simulink model "prototype_dashboard"  (R2024b)
settings: Solver=FixedStepAuto  StartTime=0.0  StopTime=inf  RelTol=1e-3  EnableMultiTasking=on
libraries: stm32f4xxblockslib x7, simulink x2
settings Model: STM32="{\"DigitalPortRead\":[{\"ID\":\"stm32test:431\"},{\"ID\":\"stm32test:432\"},{\"ID\":\"stm32test:483\"},{\"ID\":\"stm32test:484\"},{\"ID\":\"stm32test:504\"},{\"ID\":\"stm32test:505\"},{\"ID\":\"stm32test:895\"},{\"ID\":\"stm32test:896\"},{\"ID\":\"stm32test:1060\"},{\"ID\":\"stm32test:1031\"},{\"ID\":\"stm32test:1185\"},{\"ID\":\"stm32test:1186\"},{\"ID\":\"stm32test:1192\"},{\"ID\":\"stm32test:1193\"},{\"ID\":\"stm32test:1194\"},{\"ID\":\"stm32test:1195\"},{\"ID\":\"stm32test:1388:438\"},{\"ID\":\"stm32test:1590\"}],\"PWMOutput\":[{\"ID\":\"stm32test:6\"},{\"ID\":\"stm32test:8\"},{\"ID\":\"stm32test:1305\"},{\"ID\":\"stm32test:1306\"},{\"ID\":\"stm32test:1562\"}],\"DigitalPortWrite\":[{\"ID\":\"stm32test:1295\"},{\"ID\":\"stm32test:1307\"},{\"ID\":\"stm32test:1481\"},{\"ID\":\"stm32test:1482\"}],\"TimerCapture\":[{\"ID\":\"stm32test:166\"},{\"ID\":\"stm32test:836\"},{\"ID\":\"stm32test:1074\"},{\"ID\":\"stm32test:1045\"},{\"ID\":\"stm32test:1103\"},{\"ID\":\"stm32test:1388:414\"},{\"ID\":\"stm32test:1132\"},{\"ID\":\"stm32test:1468:414\"},{\"ID\":\"stm32test:1542\"}],\"HardwareInterrupt\":[{\"ID\":\"stm32test:102\"},{\"ID\":\"stm32test:1388:418\"}]}"  Creator=Tarsoly  LastModifiedBy=Asus
settings OptimizationCC: BlockReduction=off  BooleanDataType=off  EnhancedBackFolding=on  PassReuseOutputArgsAs=Individual arguments  ZeroExternalMemoryAtStartup=off  ZeroInternalMemoryAtStartup=off  MaxStackSize=512  OptimizeBlockOrder=speed  DifferentSizesBufferReuse=on  OptimizationCustomize=off  EfficientTunableParamExpr=on
settings DebuggingCC: SaveWithParameterizedLinksMsg=none  MergeDetectMultiDrivingBlocksExec=none  SignalResolutionControl=TryResolveAllWithWarning  ParameterTunabilityLossMsg=error
settings HardwareCC: ProdBitPerPointer=32  ProdBitPerSizeT=32  ProdBitPerPtrDiffT=32  ProdLargestAtomicInteger=Long  ProdLargestAtomicFloat=Double  ProdWordSize=32  ProdHWDeviceType=ARM Compatible->ARM Cortex-M  TargetLargestAtomicInteger=Long  TargetLargestAtomicFloat=Double  TargetIntDivRoundTo=Zero  TargetEndianess=LittleEndian  TargetHWDeviceType=ARM Compatible->ARM Cortex-M
settings ModelReferenceCC: PropagateSignalLabelsOutOfModel=off
settings SFSimCC: SimCustomHeaderCode="#include \"SensorActuator.h\""  SimCustomInitializer=Timer_Init_Custom();  SimUserSources=SensorActuator.c  SimUserDefines=STM32F411xE  MATLABDynamicMemAlloc=off
settings SFSimCC: SimUserIncludeDirs=|
  | D:\BME\Hetedik_felev\Szakdoga\Matlab\C_kod
  | D:\CubeMXProjectFiles\tanfolyamrobot\Core\Inc
  | D:\CubeMXProjectFiles\tanfolyamrobot\Drivers\STM32F4xx_HAL_Driver\Inc
  | D:\CubeMXProjectFiles\tanfolyamrobot\Drivers\CMSIS\Device\ST\STM32F4xx\Include
  | D:\CubeMXProjectFiles\tanfolyamrobot\Drivers\CMSIS\Include
settings RTWCC: Description=Embedded Coder  SystemTargetFile=ert.tlc  HardwareBoard=STM32F4xx Based  TemplateMakefile=ert_default_tmf  RTWUseSimCustomCode=on  CustomHeaderCode="#include \"SensorActuator.h\""  CustomSource=SensorActuator.c  CustomDefine=STM32F411xE  CustomInitializer=Timer_Init_Custom();  Toolchain=GNU Tools for ARM Embedded Processors
settings RTWCC: CustomInclude=|
  | D:\BME\Hetedik_felev\Szakdoga\Matlab\C_kod
  | D:\CubeMXProjectFiles\tanfolyamrobot\Core\Inc
  | D:\CubeMXProjectFiles\tanfolyamrobot\Drivers\STM32F4xx_HAL_Driver\Inc
  | D:\CubeMXProjectFiles\tanfolyamrobot\Drivers\CMSIS\Device\ST\STM32F4xx\Include
  | D:\CubeMXProjectFiles\tanfolyamrobot\Drivers\CMSIS\Include
settings CodeAppCC: ForceParamTrailComments=on  IgnoreCustomStorageClasses=off  OperatorAnnotations=on  SimulinkDataObjDesc=on  SFDataObjDesc=on  InsertBlockDesc=on
settings ERTTargetCC: TargetLangStandard=C99 (ISO)  CodeReplacementLibrary=ARM Cortex-M  ExtModeTransport=3  ExtModeStaticAlloc=on  ExtModeStaticAllocSize=2048  ExtModeMexFile=ext_xcp  ExtModeIntrfLevel=Level2 - Open  InlinedParameterPlacement=Hierarchical

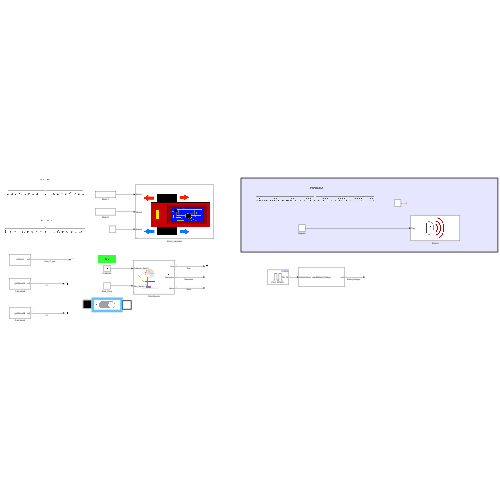
[thumbnail: Simulink's stored preview of the top-level diagram]
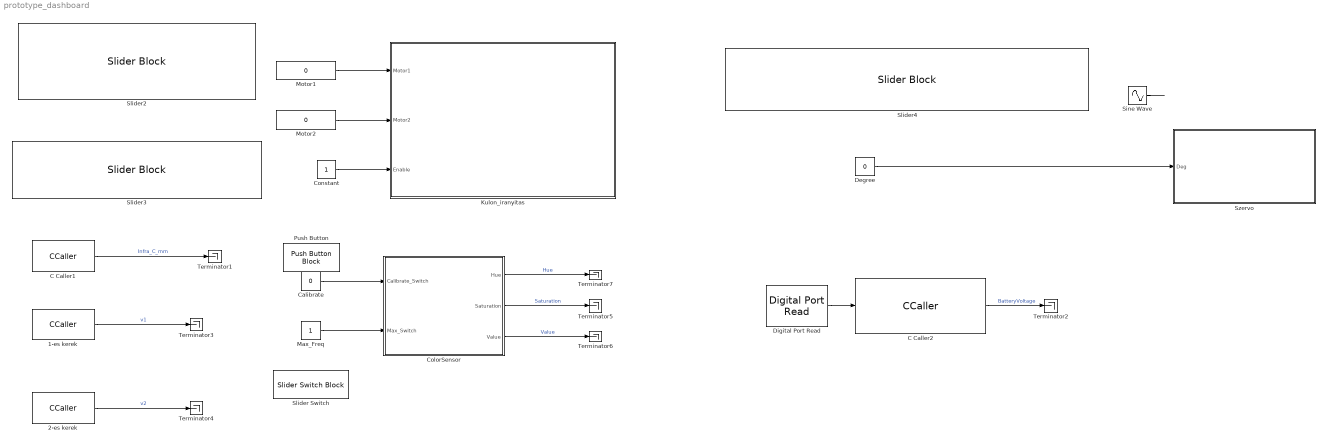
== system prototype_dashboard ==
  1-es kerek : CCaller  FunctionName=getSpeedA  PortSpecificationStruct="%)30     .    & (   8    (     @         %    \"     $    !     0         %  0 \"0    $    _    07)G3F%M90  4&]R=$YA;64 4V-O<&4     26YD97@     5'EP90      4VEZ90      27-';&]B86P   X    P    !@    @    $          4    (     0    ,    !         !   P!O=70 #@   #     &    \"     0         !0    @    !     P    $         $  # &]U=  .    .     8    (    !          %    \"     $    &     0         0    !@   $]U='!U=   #@   #@    &    \"     8         !0    @    !     0    $         \"0    @               X    X    !@    @    $          4    (     0    8    !         !     &    9&]U8FQE   .    ,     8    (    !          %    \"     $    !     0         0  $ ,0    X    P    !@    @    ) @        4    (     0    $    !          (  0"  SampleTime=0.02
  2-es kerek : CCaller  FunctionName=getSpeedB  PortSpecificationStruct="%)30     .    & (   8    (     @         %    \"     $    !     0         %  0 \"0    $    _    07)G3F%M90  4&]R=$YA;64 4V-O<&4     26YD97@     5'EP90      4VEZ90      27-';&]B86P   X    P    !@    @    $          4    (     0    ,    !         !   P!O=70 #@   #     &    \"     0         !0    @    !     P    $         $  # &]U=  .    .     8    (    !          %    \"     $    &     0         0    !@   $]U='!U=   #@   #@    &    \"     8         !0    @    !     0    $         \"0    @               X    X    !@    @    $          4    (     0    8    !         !     &    9&]U8FQE   .    ,     8    (    !          %    \"     $    !     0         0  $ ,0    X    P    !@    @    ) @        4    (     0    $    !          (  0"  SampleTime=0.02
  C Caller1 : CCaller  FunctionName=infrared  PortSpecificationStruct="%)30     .    & (   8    (     @         %    \"     $    !     0         %  0 \"0    $    _    07)G3F%M90  4&]R=$YA;64 4V-O<&4     26YD97@     5'EP90      4VEZ90      27-';&]B86P   X    P    !@    @    $          4    (     0    ,    !         !   P!O=70 #@   #     &    \"     0         !0    @    !     P    $         $  # &]U=  .    .     8    (    !          %    \"     $    &     0         0    !@   $]U='!U=   #@   #@    &    \"     8         !0    @    !     0    $         \"0    @               X    X    !@    @    $          4    (     0    8    !         !     &    =6EN=#,R   .    ,     8    (    !          %    \"     $    !     0         0  $ ,0    X    P    !@    @    ) @        4    (     0    $    !          (  0"  SampleTime=0.02
  C Caller2 : CCaller  FunctionName=readBatteryVoltage  PortSpecificationStruct="%)30     .    V ,   8    (     @         %    \"     (    !     0         %  0 \"0    $    _    07)G3F%M90  4&]R=$YA;64 4V-O<&4     26YD97@     5'EP90      4VEZ90      27-';&]B86P   X    P    !@    @    $          4    (     0    ,    !         !   P!O=70 #@   #     &    \"     0         !0    @    !     P    $         $  # &]U=  .    .     8    (    !          %    \"     $    &     0         0    !@   $]U='!U=   #@   #@    &    \"     8         !0    @    !     0    $         \"0    @               X    X    !@    @    $          4    (     0    8    !         !     &    =6EN=#$V   .    ,     8    (    !          %    \"     $    !     0         0  $ ,0    X    P    !@    @    ) @        4    (     0    $    !          (  0      #@   $     &    \"     0         !0    @    !    \"P    $         $     L   !B=71T;VY686QU90      #@   $     &    \"     0         !0    @    !    \"P    $         $     L   !B=71T;VY686QU90      #@   #@    &    \"     0         !0    @    !    !0    $         $     4   !);G!U=     X    X    !@    @    &          4    (     0    $    !          D    (               .    .     8    (    !          %    \"     $    '     0         0    !P   &)O;VQE86X #@   #     &    \"     0         !0    @    !     0    $         $  ! #$    .    ,     8    (    \"0(        %    \"     $    !     0         \"  $"  SampleTime=1
  Calibrate : Constant  Value=0
  ColorSensor : Subsystem
      mask DialogControl DescTextVar Prompt: This subsystem is for measuring the color of the ground beneath the robot.
      mask Display: image('Mask5_szin2.png', [20,20,20,20,100,100]);
  Constant : Constant
  Degree : Constant  Value=0
  Digital Port Read : stm32f4xxblockslib/Digital Port Read  PortName=GPIOA  PinNumber=[15]  ReadOperation=on  IOAsArray=off  SampleTime=1  EnableSimPort=off  hoistedMaskSrc=ECSoC/ECSimCodegen/Digital Port Read
  Kulon_iranyitas : Subsystem
      mask DialogControl Control2 Prompt: This block is meant for when you want to control the wheels independent of eachother. It can control the wheels with (-99;99) signals.
      mask Display: image('Maszk4_kulon_kerek.png', [25,25,5,0,100,100]);
  Max_Freq : Constant
  Motor1 : Constant  Value=0
  Motor2 : Constant  Value=0
  Push Button : PushButtonBlock  ButtonText=Calibrate  OffValue=0.000000
  Sine Wave : Sin  Amplitude=90  Frequency=pi  SampleTime=0.02
  Slider Switch : SliderSwitchBlock  LabelPosition=Hide
      settings: Values={{'Off', 'On'}, [0 1]}
  Slider2 : SliderBlock  ScaleMin=-99  ScaleMax=99
  Slider3 : SliderBlock  ScaleMin=-99  ScaleMax=99
  Slider4 : SliderBlock  ScaleMin=-90  ScaleMax=90
  Szervo : Subsystem
      mask Display: image('Mask6_Szervo.png', [30,10,30,10,100,100]);
  Terminator{1..7} (7 alike) : Terminator
  wires:
  Constant/1 -> Kulon_iranyitas/3(Enable)
  Motor1/1 -> Kulon_iranyitas/1(Motor1)
  Motor2/1 -> Kulon_iranyitas/2(Motor2)
  C Caller1/1 -> Terminator1/1  "Infra_C_mm"
  C Caller2/1 -> Terminator2/1  "BatteryVoltage"
  Digital Port Read/1 -> C Caller2/1
  2-es kerek/1 -> Terminator4/1  "v2"
  1-es kerek/1 -> Terminator3/1  "v1"
  Sine Wave/1 -> ?
  ColorSensor/1(Hue) -> Terminator7/1  "Hue"
  ColorSensor/2(Saturation) -> Terminator5/1  "Saturation"
  ColorSensor/3(Value) -> Terminator6/1  "Value"
  Degree/1 -> Szervo/1(Deg)
  Calibrate/1 -> ColorSensor/1(Calibrate_Switch)
  Max_Freq/1 -> ColorSensor/2(Max_Switch)

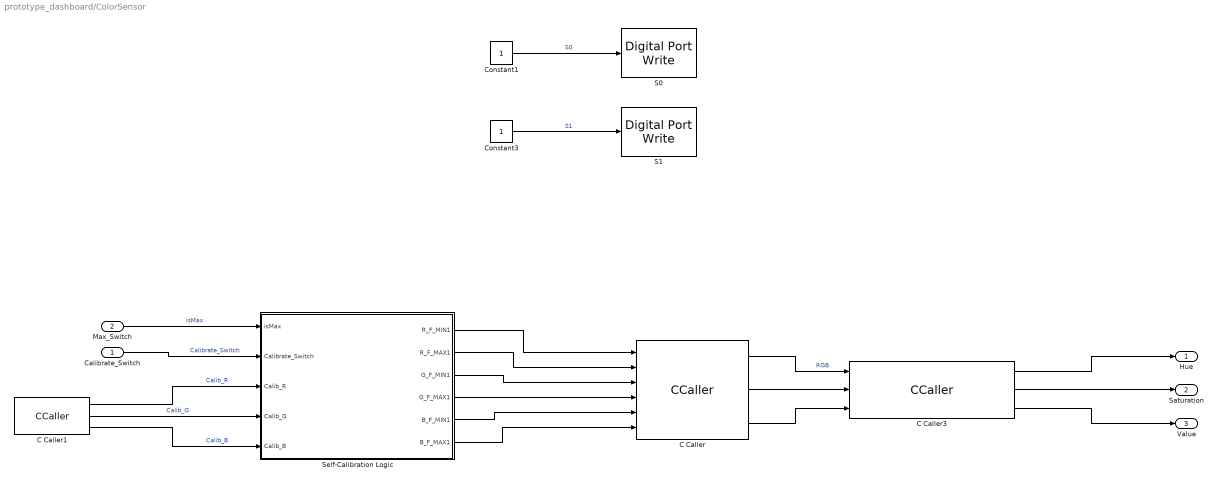
== system prototype_dashboard/ColorSensor ==
  Calibrate_Switch : Inport
  Max_Switch : Inport  Port=2
  C Caller : CCaller  FunctionName=getRGB  PortSpecificationStruct="%)30     .    > \\   8    (     @         %    \"     D    !     0         %  0 \"0    $    _    07)G3F%M90  4&]R=$YA;64 4V-O<&4     26YD97@     5'EP90      4VEZ90      27-';&]B86P   X    P    !@    @    $          4    (     0    $    !         !   0!2    #@   #     &    \"     0         !0    @    !     0    $         $  ! %(    .    .     8    (    !          %    \"     $    &     0         0  ...(+4961 chars)"  SampleTime=0.02
  C Caller1 : CCaller  FunctionName=calibrateRGB  PortSpecificationStruct="%)30     .    6 4   8    (     @         %    \"     ,    !     0         %  0 \"0    $    _    07)G3F%M90  4&]R=$YA;64 4V-O<&4     26YD97@     5'EP90      4VEZ90      27-';&]B86P   X    P    !@    @    $          4    (     0    $    !         !   0!2    #@   #     &    \"     0         !0    @    !     0    $         $  ! %(    .    .     8    (    !          %    \"     $    &     0         0    !@   $]U='!U=   #@   #@    &    \"     8         !0    @    !     0    $         \"0    @               X    X    !@    @    $          4    (     0    8    !         !     &    =6EN=#$V   .    ,     8    (    !          %    \"     $    !     0         0  $ ,0    X    P    !@    @    ) @        4    (     0    $    !          (  0      #@   #     &    \"     0         !0    @    !     0    $         $  ! $<    .    ,     8    (    !          %    \"     $    !     0         0  $ 1P    X    X    !@    @    $          4    (     0    8    !         !     &    3W5T<'5T   .    .     8    (    !@         %    \"     $    !     0         )    \"            / _#@   #@    &    \"     0         !0    @    !    !@    $         $     8   !U:6YT,38   X    P    !@    @    $          4    (     0    $    !         !   0 Q    #@   #     &    \"     D\"        !0    @    !     0    $          @ !       .    ,     8    (    !          %    \"     $    !     0         0  $ 0@    X    P    !@    @    $          4    (     0    $    !         !   0!\"    #@   #@    &    \"     0         !0    @    !    !@    $         $     8   !/=71P=70   X    X    !@    @    &          4    (     0    $    !          D    (             $ .    .     8    (    !          %    \"     $    &     0         0    !@   '5I;G0Q-@  #@   #     &    \"     0         !0    @    !     0    $         $  ! #$    .    ,     8    (    \"0(        %    \"     $    !     0         \"  $"  SampleTime=0.02
  C Caller3 : CCaller  FunctionName=getHSVfromRGB  PortSpecificationStruct="%)30     .    : H   8    (     @         %    \"     8    !     0         %  0 \"0    $    _    07)G3F%M90  4&]R=$YA;64 4V-O<&4     26YD97@     5'EP90      4VEZ90      27-';&]B86P   X    P    !@    @    $          4    (     0    $    !         !   0!2    #@   #     &    \"     0         !0    @    !     0    $         $  ! %(    .    .     8    (    !          %    \"     $    %     0         0   ...(+3211 chars)"
  Constant1 : Constant
  Constant3 : Constant
  S0 : stm32f4xxblockslib/Digital Port Write  PortName=GPIOC  PinNumber=[12]  ReadOperation=off  IOAsArray=on  EnableSimPort=off  hoistedMaskSrc=ECSoC/ECSimCodegen/Digital Port Write
  S1 : stm32f4xxblockslib/Digital Port Write  PortName=GPIOD  PinNumber=[2]  ReadOperation=off  IOAsArray=on  EnableSimPort=off  hoistedMaskSrc=ECSoC/ECSimCodegen/Digital Port Write
  Self-Calibration Logic : Subsystem
  Hue : Outport
  Saturation : Outport  Port=2
  Value : Outport  Port=3
  wires:
  Constant3/1 -> S1/1  "S1"
  Constant1/1 -> S0/1  "S0"
  C Caller3/1 -> Hue/1
  C Caller3/2 -> Saturation/1
  C Caller3/3 -> Value/1
  C Caller/1 -> C Caller3/1  "RGB"
  C Caller/2 -> C Caller3/2
  C Caller/3 -> C Caller3/3
  Max_Switch/1 -> Self-Calibration Logic/1(isMax)  "isMax"
  Calibrate_Switch/1 -> Self-Calibration Logic/2(Calibrate_Switch)  "Calibrate_Switch"
  C Caller1/1 -> Self-Calibration Logic/3(Calib_R)  "Calib_R"
  C Caller1/2 -> Self-Calibration Logic/4(Calib_G)  "Calib_G"
  C Caller1/3 -> Self-Calibration Logic/5(Calib_B)  "Calib_B"
  Self-Calibration Logic/1(R_F_MIN1) -> C Caller/1
  Self-Calibration Logic/2(R_F_MAX1) -> C Caller/2
  Self-Calibration Logic/3(G_F_MIN1) -> C Caller/3
  Self-Calibration Logic/4(G_F_MAX1) -> C Caller/4
  Self-Calibration Logic/5(B_F_MIN1) -> C Caller/5
  Self-Calibration Logic/6(B_F_MAX1) -> C Caller/6

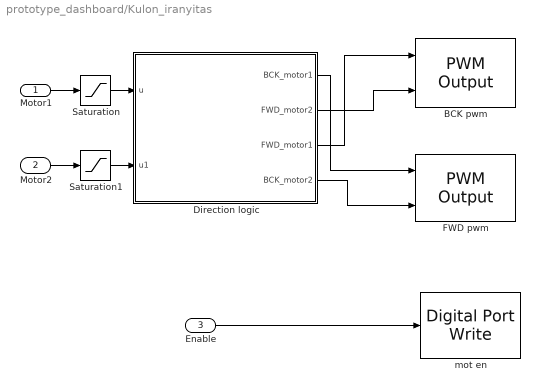
== system prototype_dashboard/Kulon_iranyitas ==
  Motor1 : Inport
  Motor2 : Inport  Port=2
  Enable : Inport  Port=3
  BCK pwm : stm32f4xxblockslib/PWM Output  TimerModule=TIM1  DutycycleUnits=Percentage  EnableChannel1=on  EnableChannel2=on  EnableChannel3=off  EnableChannel4=off  EnableCounterInput=off  EnableMainOutputInput=off  EnableFrequencyInput=off  SetRCAfterCE=off  OutputDirection=off  OutputMainOutputEnableStatus=off  SampleTime=0.1  EnableSimPort=off  EnableUpdateEvent=off  EnableCaptureCompare1Event=off  EnableCaptureCompare2Event=off  EnableCaptureCompare3Event=off  EnableCaptureCompare4Event=off  EnableTriggerEvent=off  EnableBreakEvent=off  ProcessorFamily=STM32F4  hoistedMaskSrc=ECSoC/ECSimCodegen/PWM Output
  Direction logic : Subsystem
  "FWD pwm " : stm32f4xxblockslib/PWM Output  TimerModule=TIM3  DutycycleUnits=Percentage  EnableChannel1=off  EnableChannel2=off  EnableChannel3=on  EnableChannel4=on  EnableCounterInput=off  EnableMainOutputInput=off  EnableFrequencyInput=off  SetRCAfterCE=off  OutputDirection=off  OutputMainOutputEnableStatus=off  SampleTime=0.1  EnableSimPort=off  EnableUpdateEvent=off  EnableCaptureCompare1Event=off  EnableCaptureCompare2Event=off  EnableCaptureCompare3Event=off  EnableCaptureCompare4Event=off  EnableTriggerEvent=off  EnableBreakEvent=off  ProcessorFamily=STM32F4  hoistedMaskSrc=ECSoC/ECSimCodegen/PWM Output
  Saturation : Saturate  UpperLimit=99  LowerLimit=-99
  Saturation1 : Saturate  UpperLimit=99  LowerLimit=-99
  mot en : stm32f4xxblockslib/Digital Port Write  PortName=GPIOC  PinNumber=5  ReadOperation=off  IOAsArray=on  EnableSimPort=off  hoistedMaskSrc=ECSoC/ECSimCodegen/Digital Port Write
  wires:
  Enable/1 -> mot en/1
  Motor1/1 -> Saturation/1
  Motor2/1 -> Saturation1/1
  Direction logic/1(BCK_motor1) -> "FWD pwm "/1
  Direction logic/2(FWD_motor2) -> BCK pwm/2
  Direction logic/3(FWD_motor1) -> BCK pwm/1
  Direction logic/4(BCK_motor2) -> "FWD pwm "/2
  Saturation/1 -> Direction logic/1(u)
  Saturation1/1 -> Direction logic/2(u1)

== system prototype_dashboard/Szervo ==
  Deg : Inport
  PWM Output : stm32f4xxblockslib/PWM Output  TimerModule=TIM11  DutycycleUnits=Percentage  EnableChannel1=on  EnableChannel2=off  EnableChannel3=off  EnableChannel4=off  EnableCounterInput=off  EnableMainOutputInput=off  EnableFrequencyInput=off  SetRCAfterCE=off  OutputDirection=off  OutputMainOutputEnableStatus=off  SampleTime=0.1  EnableSimPort=off  EnableUpdateEvent=off  EnableCaptureCompare1Event=off  EnableCaptureCompare2Event=off  EnableCaptureCompare3Event=off  EnableCaptureCompare4Event=off  EnableTriggerEvent=off  EnableBreakEvent=off  ProcessorFamily=STM32F4  hoistedMaskSrc=ECSoC/ECSimCodegen/PWM Output
  Subsystem2 : Subsystem
  wires:
  Subsystem2/1(f(x)) -> PWM Output/1  "percent"
  Deg/1 -> Subsystem2/1(x)  "x"

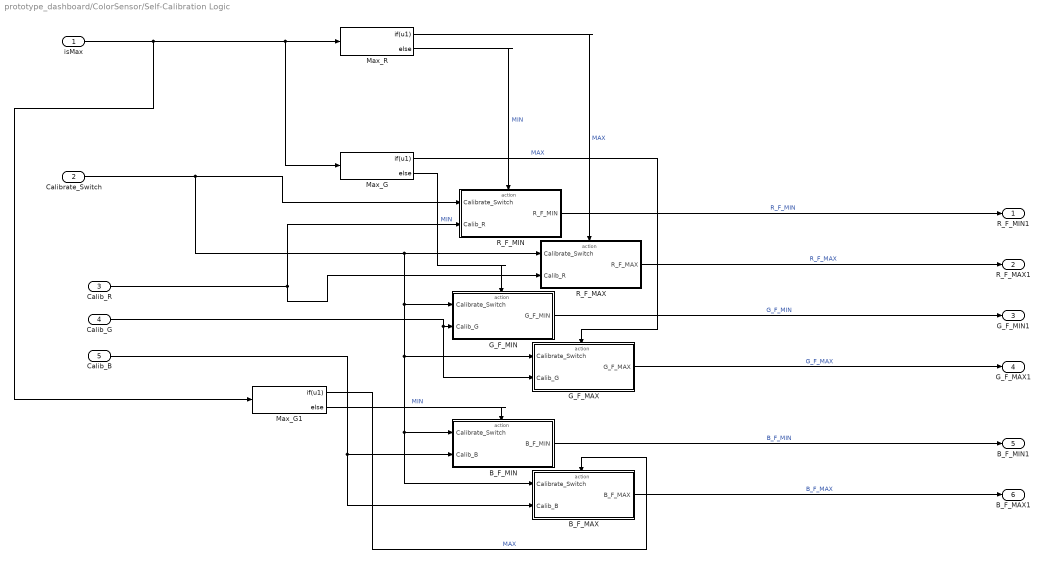
== system prototype_dashboard/ColorSensor/Self-Calibration Logic ==
  isMax : Inport
  Calibrate_Switch : Inport  Port=2
  Calib_R : Inport  Port=3
  Calib_G : Inport  Port=4
  Calib_B : Inport  Port=5
  B_F_MAX : Subsystem  TreatAsAtomicUnit=on
  B_F_MIN : Subsystem  TreatAsAtomicUnit=on
  G_F_MAX : Subsystem  TreatAsAtomicUnit=on
  G_F_MIN : Subsystem  TreatAsAtomicUnit=on
  Max_G : If  IfExpression=u1
  Max_G1 : If  IfExpression=u1
  Max_R : If  IfExpression=u1
  R_F_MAX : Subsystem  TreatAsAtomicUnit=on
  R_F_MIN : Subsystem  TreatAsAtomicUnit=on
  R_F_MIN1 : Outport
  R_F_MAX1 : Outport  Port=2
  G_F_MIN1 : Outport  Port=3
  G_F_MAX1 : Outport  Port=4
  B_F_MIN1 : Outport  Port=5
  B_F_MAX1 : Outport  Port=6
  wires:
  G_F_MIN/1(G_F_MIN) -> G_F_MIN1/1  "G_F_MIN"
  B_F_MAX/1(B_F_MAX) -> B_F_MAX1/1  "B_F_MAX"
  Calib_R/1 -> R_F_MAX/2(Calib_R), R_F_MIN/2(Calib_R)
  Calibrate_Switch/1 -> R_F_MAX/1(Calibrate_Switch), G_F_MIN/1(Calibrate_Switch), B_F_MAX/1(Calibrate_Switch), B_F_MIN/1(Calibrate_Switch), G_F_MAX/1(Calibrate_Switch), R_F_MIN/1(Calibrate_Switch)
  Max_R/1 -> R_F_MAX/Action  "MAX"
  Calib_G/1 -> G_F_MAX/2(Calib_G), G_F_MIN/2(Calib_G)
  G_F_MAX/1(G_F_MAX) -> G_F_MAX1/1  "G_F_MAX"
  Max_R/2 -> R_F_MIN/Action  "MIN"
  isMax/1 -> Max_G/1, Max_R/1, Max_G1/1
  Calib_B/1 -> B_F_MAX/2(Calib_B), B_F_MIN/2(Calib_B)
  B_F_MIN/1(B_F_MIN) -> B_F_MIN1/1  "B_F_MIN"
  R_F_MIN/1(R_F_MIN) -> R_F_MIN1/1  "R_F_MIN"
  R_F_MAX/1(R_F_MAX) -> R_F_MAX1/1  "R_F_MAX"
  Max_G/1 -> G_F_MAX/Action  "MAX"
  Max_G/2 -> G_F_MIN/Action  "MIN"
  Max_G1/1 -> B_F_MAX/Action  "MAX"
  Max_G1/2 -> B_F_MIN/Action  "MIN"

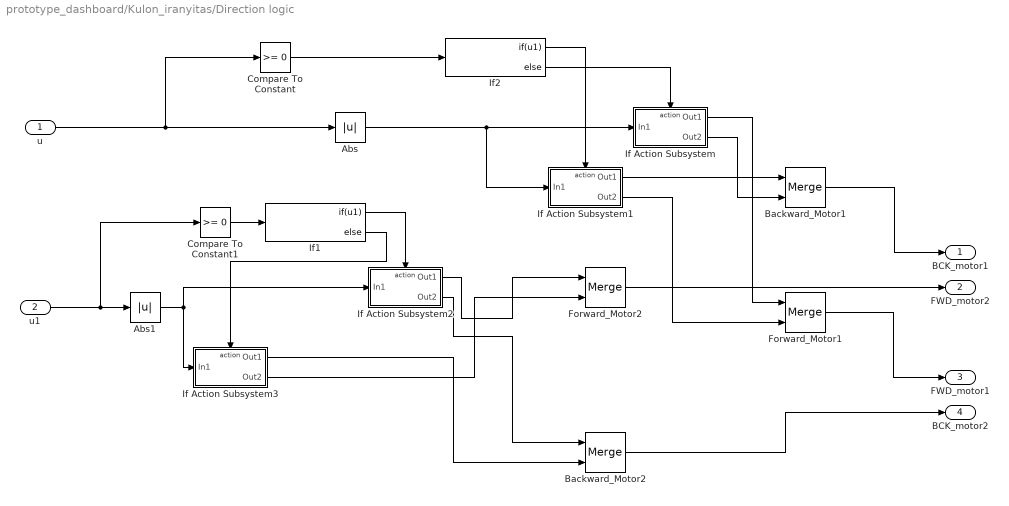
== system prototype_dashboard/Kulon_iranyitas/Direction logic ==
  u : Inport
  u1 : Inport  Port=2
  Abs : Abs  SaturateOnIntegerOverflow=off
  Abs1 : Abs  SaturateOnIntegerOverflow=off
  Backward_Motor1 : Merge
  Backward_Motor2 : Merge
  Compare To Constant : simulink/Logic and Bit Operations/Compare To Constant  relop=>=  const=0  OutDataTypeStr=boolean
  Compare To Constant1 : simulink/Logic and Bit Operations/Compare To Constant  relop=>=  const=0  OutDataTypeStr=boolean
  Forward_Motor1 : Merge
  Forward_Motor2 : Merge
  If Action Subsystem : Subsystem  TreatAsAtomicUnit=on
  If Action Subsystem1 : Subsystem  TreatAsAtomicUnit=on
  If Action Subsystem2 : Subsystem  TreatAsAtomicUnit=on
  If Action Subsystem3 : Subsystem  TreatAsAtomicUnit=on
  If1 : If  IfExpression=u1
  If2 : If  IfExpression=u1
  BCK_motor1 : Outport
  FWD_motor2 : Outport  Port=2
  FWD_motor1 : Outport  Port=3
  BCK_motor2 : Outport  Port=4
  wires:
  Forward_Motor2/1 -> FWD_motor2/1
  If Action Subsystem/1(Out1) -> Forward_Motor1/1
  If Action Subsystem1/1(Out1) -> Backward_Motor1/1
  If Action Subsystem3/2(Out2) -> Forward_Motor2/2
  Compare To Constant/1 -> If2/1
  If Action Subsystem3/1(Out1) -> Backward_Motor2/2
  Abs1/1 -> If Action Subsystem2/1(In1), If Action Subsystem3/1(In1)
  Abs/1 -> If Action Subsystem1/1(In1), If Action Subsystem/1(In1)
  If Action Subsystem/2(Out2) -> Backward_Motor1/2
  u/1 -> Abs/1, Compare To Constant/1
  Backward_Motor2/1 -> BCK_motor2/1
  If1/1 -> If Action Subsystem2/Action
  Compare To Constant1/1 -> If1/1
  u1/1 -> Compare To Constant1/1, Abs1/1
  Backward_Motor1/1 -> BCK_motor1/1
  If1/2 -> If Action Subsystem3/Action
  If Action Subsystem1/2(Out2) -> Forward_Motor1/2
  If Action Subsystem2/1(Out1) -> Forward_Motor2/1
  If Action Subsystem2/2(Out2) -> Backward_Motor2/1
  Forward_Motor1/1 -> FWD_motor1/1
  If2/2 -> If Action Subsystem/Action
  If2/1 -> If Action Subsystem1/Action

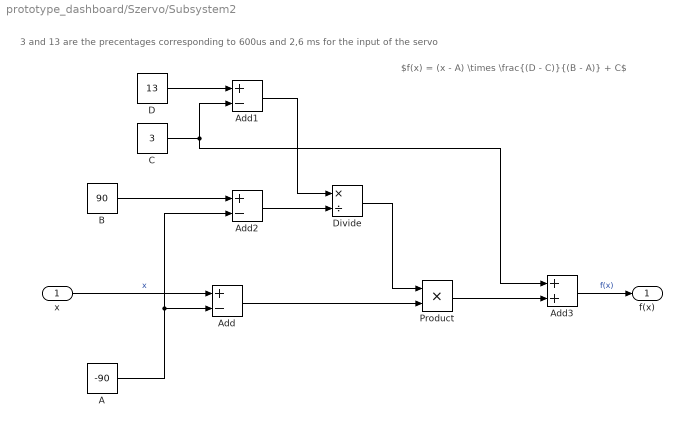
== system prototype_dashboard/Szervo/Subsystem2 ==
  note: 3 and 13 are the precentages corresponding to 600us and 2,6 ms for the input of the servo
  note: $f(x) = (x - A) \times \frac{(D - C)}{(B - A)} + C$
  x : Inport
  A : Constant  Value=-90
  Add : Sum  Inputs=+-
  Add1 : Sum  Inputs=+-
  Add2 : Sum  Inputs=+-
  Add3 : Sum
  B : Constant  Value=90
  C : Constant  Value=3
  D : Constant  Value=13
  Divide : Product  Inputs=*/
  Product : Product
  f(x) : Outport
  wires:
  x/1 -> Add/1  "x"
  A/1 -> Add2/2, Add/2
  Add/1 -> Product/2
  D/1 -> Add1/1
  C/1 -> Add1/2, Add3/1
  Add1/1 -> Divide/1
  Add2/1 -> Divide/2
  B/1 -> Add2/1
  Product/1 -> Add3/2
  Add3/1 -> f(x)/1  "f(x)"
  Divide/1 -> Product/1

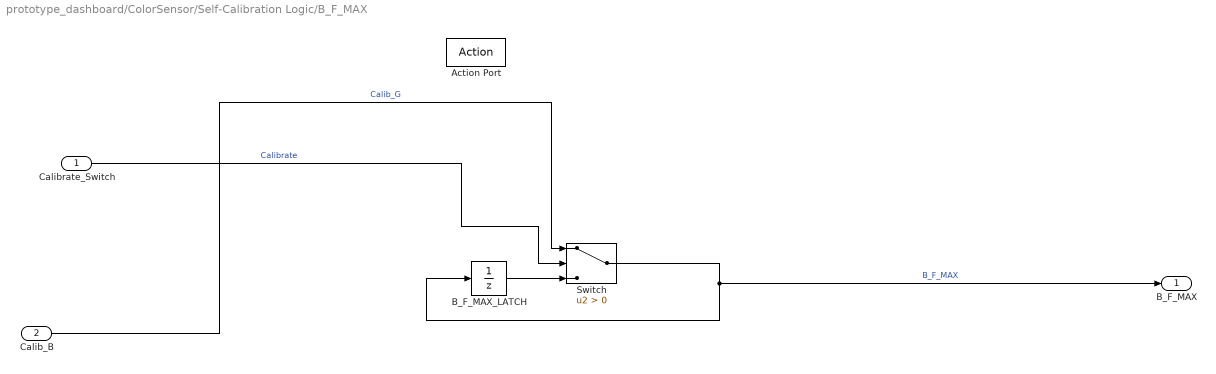
== system prototype_dashboard/ColorSensor/Self-Calibration Logic/B_F_MAX ==
  Calibrate_Switch : Inport
  Calib_B : Inport  Port=2
  Action Port : ActionPort  ActionPortLabel=if(u1)
  B_F_MAX_LATCH : UnitDelay  InitialCondition=18200  SampleTime=-1  HasFrameUpgradeWarning=on
  Switch : Switch  Criteria=u2 > Threshold  SaturateOnIntegerOverflow=off  InputSameDT=off
  B_F_MAX : Outport
  wires:
  Calibrate_Switch/1 -> Switch/2  "Calibrate"
  Calib_B/1 -> Switch/1  "Calib_G"
  Switch/1 -> B_F_MAX_LATCH/1, B_F_MAX/1  "B_F_MAX"
  B_F_MAX_LATCH/1 -> Switch/3

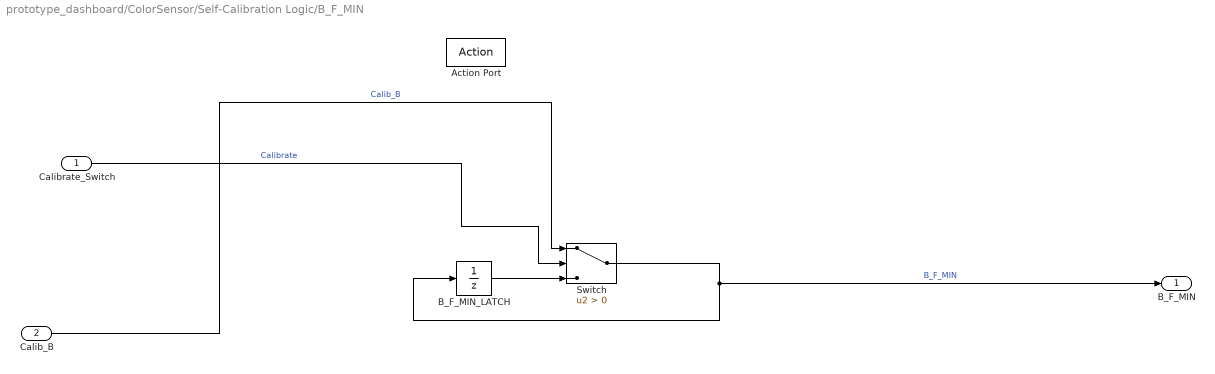
== system prototype_dashboard/ColorSensor/Self-Calibration Logic/B_F_MIN ==
  Calibrate_Switch : Inport
  Calib_B : Inport  Port=2
  Action Port : ActionPort  ActionPortLabel=else
  B_F_MIN_LATCH : UnitDelay  InitialCondition=3200  SampleTime=-1  HasFrameUpgradeWarning=on
  Switch : Switch  Criteria=u2 > Threshold  SaturateOnIntegerOverflow=off  InputSameDT=off
  B_F_MIN : Outport
  wires:
  Calibrate_Switch/1 -> Switch/2  "Calibrate"
  Calib_B/1 -> Switch/1  "Calib_B"
  Switch/1 -> B_F_MIN_LATCH/1, B_F_MIN/1  "B_F_MIN"
  B_F_MIN_LATCH/1 -> Switch/3

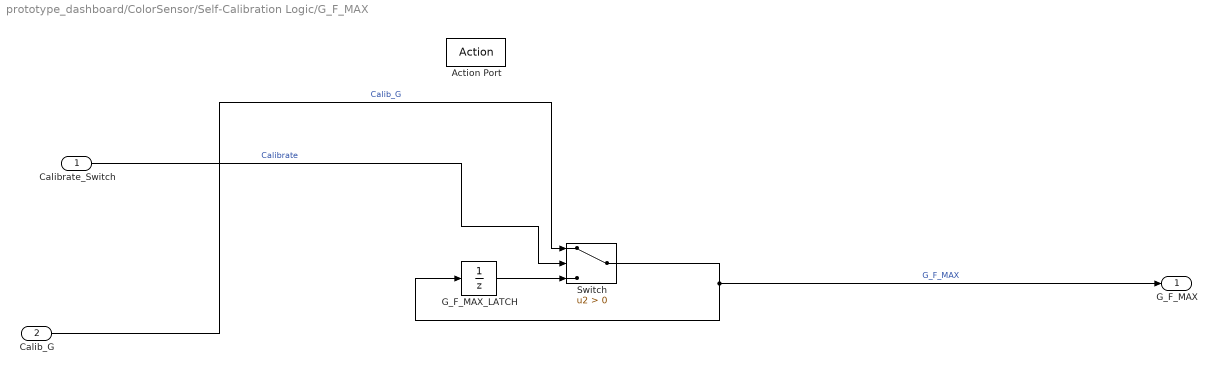
== system prototype_dashboard/ColorSensor/Self-Calibration Logic/G_F_MAX ==
  Calibrate_Switch : Inport
  Calib_G : Inport  Port=2
  Action Port : ActionPort  ActionPortLabel=if(u1)
  G_F_MAX_LATCH : UnitDelay  InitialCondition=16700  SampleTime=-1  HasFrameUpgradeWarning=on
  Switch : Switch  Criteria=u2 > Threshold  SaturateOnIntegerOverflow=off  InputSameDT=off
  G_F_MAX : Outport
  wires:
  Calibrate_Switch/1 -> Switch/2  "Calibrate"
  Calib_G/1 -> Switch/1  "Calib_G"
  Switch/1 -> G_F_MAX_LATCH/1, G_F_MAX/1  "G_F_MAX"
  G_F_MAX_LATCH/1 -> Switch/3

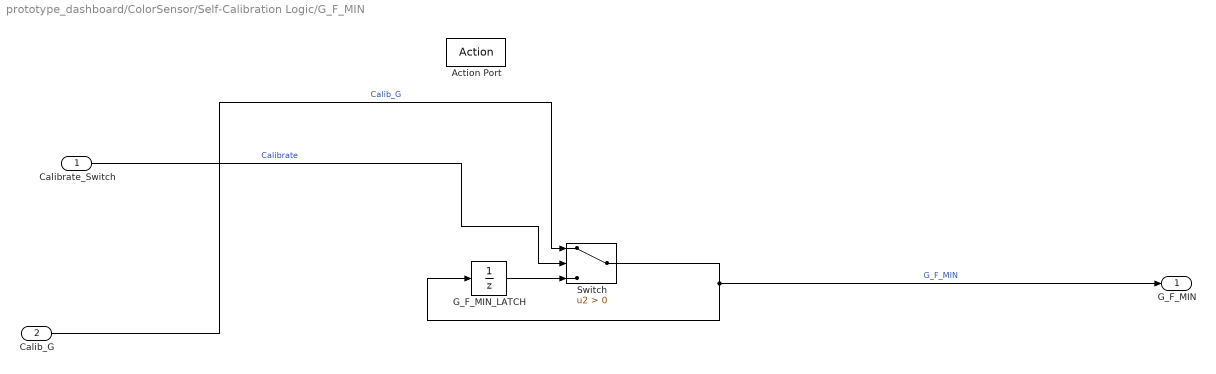
== system prototype_dashboard/ColorSensor/Self-Calibration Logic/G_F_MIN ==
  Calibrate_Switch : Inport
  Calib_G : Inport  Port=2
  Action Port : ActionPort  ActionPortLabel=else
  G_F_MIN_LATCH : UnitDelay  InitialCondition=3200  SampleTime=-1  HasFrameUpgradeWarning=on
  Switch : Switch  Criteria=u2 > Threshold  SaturateOnIntegerOverflow=off  InputSameDT=off
  G_F_MIN : Outport
  wires:
  Calibrate_Switch/1 -> Switch/2  "Calibrate"
  Calib_G/1 -> Switch/1  "Calib_G"
  Switch/1 -> G_F_MIN_LATCH/1, G_F_MIN/1  "G_F_MIN"
  G_F_MIN_LATCH/1 -> Switch/3

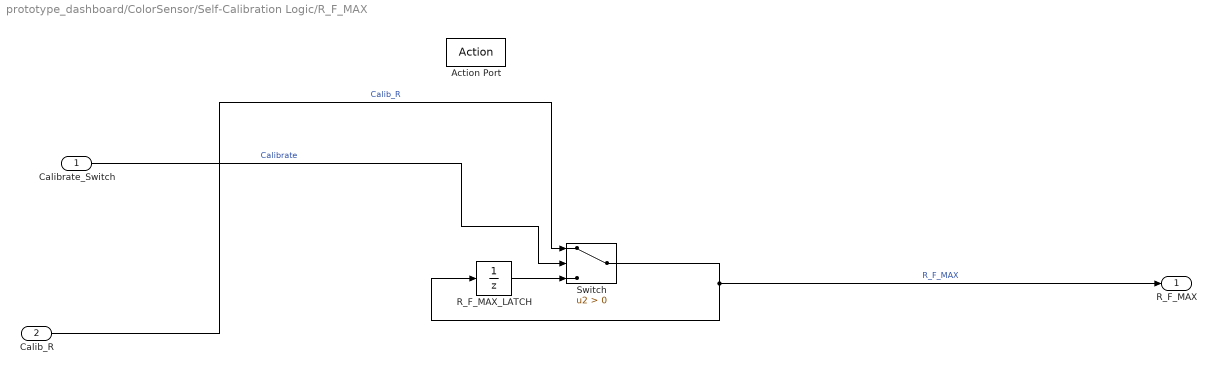
== system prototype_dashboard/ColorSensor/Self-Calibration Logic/R_F_MAX ==
  Calibrate_Switch : Inport
  Calib_R : Inport  Port=2
  Action Port : ActionPort  ActionPortLabel=if(u1)
  R_F_MAX_LATCH : UnitDelay  InitialCondition=23200  SampleTime=-1  HasFrameUpgradeWarning=on
  Switch : Switch  Criteria=u2 > Threshold  SaturateOnIntegerOverflow=off  InputSameDT=off
  R_F_MAX : Outport
  wires:
  Calibrate_Switch/1 -> Switch/2  "Calibrate"
  Calib_R/1 -> Switch/1  "Calib_R"
  Switch/1 -> R_F_MAX_LATCH/1, R_F_MAX/1  "R_F_MAX"
  R_F_MAX_LATCH/1 -> Switch/3

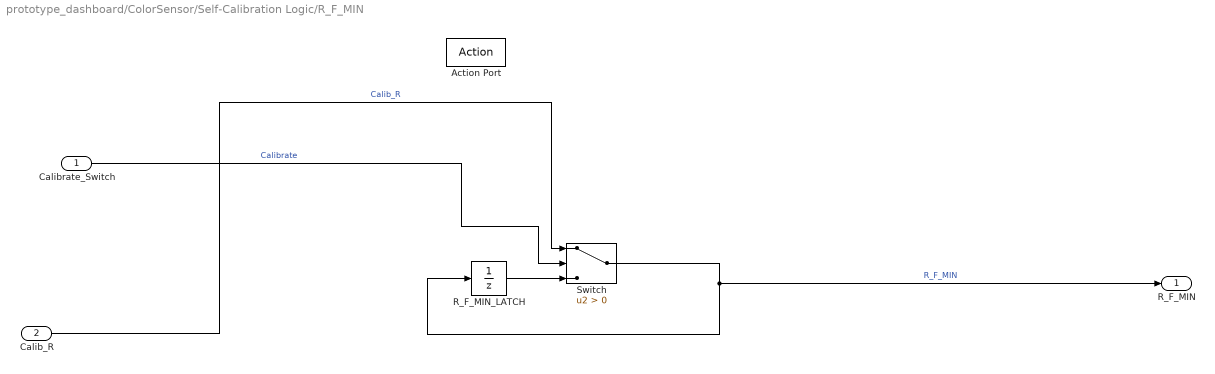
== system prototype_dashboard/ColorSensor/Self-Calibration Logic/R_F_MIN ==
  Calibrate_Switch : Inport
  Calib_R : Inport  Port=2
  Action Port : ActionPort  ActionPortLabel=else
  R_F_MIN_LATCH : UnitDelay  InitialCondition=5100  SampleTime=-1  HasFrameUpgradeWarning=on
  Switch : Switch  Criteria=u2 > Threshold  SaturateOnIntegerOverflow=off  InputSameDT=off
  R_F_MIN : Outport
  wires:
  Calibrate_Switch/1 -> Switch/2  "Calibrate"
  Calib_R/1 -> Switch/1  "Calib_R"
  Switch/1 -> R_F_MIN_LATCH/1, R_F_MIN/1  "R_F_MIN"
  R_F_MIN_LATCH/1 -> Switch/3

== system prototype_dashboard/Kulon_iranyitas/Direction logic/If Action Subsystem ==
  In1 : Inport
  Action Port : ActionPort  ActionPortLabel=else
  Constant : Constant  Value=0
  Out1 : Outport
  Out2 : Outport  Port=2
  wires:
  In1/1 -> Out1/1
  Constant/1 -> Out2/1

== system prototype_dashboard/Kulon_iranyitas/Direction logic/If Action Subsystem1 ==
  In1 : Inport
  Action Port : ActionPort  ActionPortLabel=if(u1)
  Constant : Constant  Value=0
  Out1 : Outport
  Out2 : Outport  Port=2
  wires:
  In1/1 -> Out1/1
  Constant/1 -> Out2/1

== system prototype_dashboard/Kulon_iranyitas/Direction logic/If Action Subsystem2 ==
  In1 : Inport
  Action Port : ActionPort  ActionPortLabel=if(u1)
  Constant : Constant  Value=0
  Out1 : Outport
  Out2 : Outport  Port=2
  wires:
  In1/1 -> Out1/1
  Constant/1 -> Out2/1

== system prototype_dashboard/Kulon_iranyitas/Direction logic/If Action Subsystem3 ==
  In1 : Inport
  Action Port : ActionPort  ActionPortLabel=else
  Constant : Constant  Value=0
  Out1 : Outport
  Out2 : Outport  Port=2
  wires:
  In1/1 -> Out1/1
  Constant/1 -> Out2/1
